simulink model "FLIGHT_Hexacopter_V2_1"  (R2024a)
settings: Solver=FixedStepDiscrete  StartTime=0.0  StopTime=inf  FixedStep=SampleTime_SAS  RelTol=1e-3  EnableMultiTasking=on
InitFcn:
  | Init_FLIGHT_Hexacopter
values from neighbouring files (symbols this model uses):
  d2r = pi/180    (= 0.0174532925199)    [Init_FLIGHT_Hexacopter.m]
  Jxx = 0.0211    [Init_FLIGHT_Hexacopter.m]
  Jyy = 0.0219    [Init_FLIGHT_Hexacopter.m]
  Jzz = 0.0366    [Init_FLIGHT_Hexacopter.m]
  Kpp = 3.3894    [Init_FLIGHT_Hexacopter_fromNCMS.m]
  Kpr = 3.3894    [Init_FLIGHT_Hexacopter_fromNCMS.m]
  MAX_CONTROL_ANGLE_PITCH = 30*pi/180    (= 0.523598775598)    [Init_FLIGHT_Hexacopter.m]    (also in Init_FLIGHT_Hexacopter_fromNCMS.m = 0.349065850399)
  MAX_CONTROL_ANGLE_RATE_PITCH = 360*pi/180    (= 6.28318530718)    [Init_FLIGHT_Hexacopter.m]    (also in Init_FLIGHT_Hexacopter_fromNCMS.m)
  MAX_CONTROL_ANGLE_RATE_ROLL = 360*pi/180    (= 6.28318530718)    [Init_FLIGHT_Hexacopter.m]    (also in Init_FLIGHT_Hexacopter_fromNCMS.m)
  MAX_CONTROL_ANGLE_RATE_Y = 120*pi/180    (= 2.09439510239)    [Init_FLIGHT_Hexacopter.m]    (also in Init_FLIGHT_Hexacopter_fromNCMS.m)
  MAX_CONTROL_ANGLE_ROLL = 30*pi/180    (= 0.523598775598)    [Init_FLIGHT_Hexacopter.m]    (also in Init_FLIGHT_Hexacopter_fromNCMS.m = 0.349065850399)
  MAX_CONTROL_VELOCITY_XY = 1.5    [Init_FLIGHT_Hexacopter.m]    (also in Init_FLIGHT_Hexacopter_fromNCMS.m)
  MAX_CONTROL_VELOCITY_Z = 1    [Init_FLIGHT_Hexacopter.m]    (also in Init_FLIGHT_Hexacopter_fromNCMS.m)
  SampleTime = 1/250    (= 0.004)    [Init_FLIGHT_Hexacopter.m]    (also in Init_FLIGHT_Hexacopter_fromNCMS.m = 0.01)
  SampleTime_SAS = 1/1000    (= 0.001)    [Init_FLIGHT_Hexacopter.m]
undefined symbols (not defined in the file or in its folder): arguments, DiscIntNeverNeededParam, event_sequence, id, log_levels, MPC_Z_D, MPC_Z_I, MPC_Z_P, timestamp
libraries: px4lib x42, simulink x9, px4Utilslib x8, px4uORBlib x8, slpidlib x5, simulink_extras x2, sharedtransform x1, px4Sensorslib x1, matrix_library x1
(part 2 of 3)

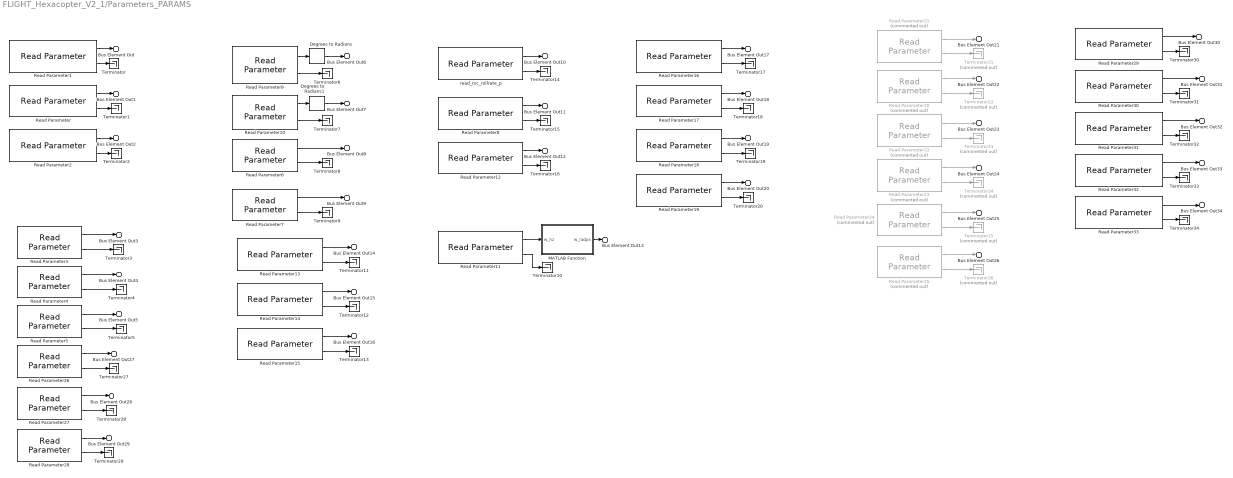
== system FLIGHT_Hexacopter_V2_1/Parameters_PARAMS ==
  Degrees to Radians : simulink_extras/Transformations/Degrees to Radians
  Degrees to Radians1 : simulink_extras/Transformations/Degrees to Radians
  MATLAB Function : MATLAB Function  TreatAsAtomicUnit=on
  Read Parameter : px4lib/Read Parameter  ParameterName=DOUBLET_DT  DataType=FLOAT  SampleTime=SampleTime
      settings: SourceProductName=UAV Toolbox Support Package for PX4 Autopilots
  Read Parameter1 : px4lib/Read Parameter  ParameterName=DOUBLET_PEAK_ANG  DataType=FLOAT  SampleTime=SampleTime
      settings: SourceProductName=UAV Toolbox Support Package for PX4 Autopilots
  Read Parameter10 : px4lib/Read Parameter  ParameterName=MC_PITCHRATE_MAX  DataType=FLOAT  SampleTime=SampleTime
      settings: SourceProductName=UAV Toolbox Support Package for PX4 Autopilots
  Read Parameter11 : px4lib/Read Parameter  ParameterName=IMU_DGYRO_CUTOFF  DataType=FLOAT  SampleTime=SampleTime
      settings: SourceProductName=UAV Toolbox Support Package for PX4 Autopilots
  Read Parameter12 : px4lib/Read Parameter  ParameterName=MC_ROLLRATE_D  DataType=FLOAT  SampleTime=SampleTime
      settings: SourceProductName=UAV Toolbox Support Package for PX4 Autopilots
  Read Parameter13 : px4lib/Read Parameter  ParameterName=MC_PITCHRATE_P  DataType=FLOAT  SampleTime=SampleTime
      settings: SourceProductName=UAV Toolbox Support Package for PX4 Autopilots
  Read Parameter14 : px4lib/Read Parameter  ParameterName=MC_PITCHRATE_I  DataType=FLOAT  SampleTime=SampleTime
      settings: SourceProductName=UAV Toolbox Support Package for PX4 Autopilots
  Read Parameter15 : px4lib/Read Parameter  ParameterName=MC_PITCHRATE_D  DataType=FLOAT  SampleTime=SampleTime
      settings: SourceProductName=UAV Toolbox Support Package for PX4 Autopilots
  Read Parameter16 : px4lib/Read Parameter  ParameterName=MC_YAWRATE_P  DataType=FLOAT  SampleTime=SampleTime
      settings: SourceProductName=UAV Toolbox Support Package for PX4 Autopilots
  Read Parameter17 : px4lib/Read Parameter  ParameterName=MC_YAWRATE_I  DataType=FLOAT  SampleTime=SampleTime
      settings: SourceProductName=UAV Toolbox Support Package for PX4 Autopilots
  Read Parameter18 : px4lib/Read Parameter  ParameterName=MC_YAWRATE_D  DataType=FLOAT  SampleTime=SampleTime
      settings: SourceProductName=UAV Toolbox Support Package for PX4 Autopilots
  Read Parameter19 : px4lib/Read Parameter  ParameterName=MC_YAWRATE_FF  DataType=FLOAT  SampleTime=SampleTime
      settings: SourceProductName=UAV Toolbox Support Package for PX4 Autopilots
  Read Parameter2 : px4lib/Read Parameter  ParameterName=DOUBLET_AXIS  DataType=INT32  SampleTime=SampleTime
      settings: SourceProductName=UAV Toolbox Support Package for PX4 Autopilots
  Read Parameter20 : px4lib/Read Parameter  Commented=on  ParameterName=FDD_M2_STATUS  DataType=INT32  SampleTime=SampleTime
      settings: SourceProductName=UAV Toolbox Support Package for PX4 Autopilots
  Read Parameter21 : px4lib/Read Parameter  Commented=on  ParameterName=FDD_M1_STATUS  DataType=INT32  SampleTime=SampleTime
      settings: SourceProductName=UAV Toolbox Support Package for PX4 Autopilots
  Read Parameter22 : px4lib/Read Parameter  Commented=on  ParameterName=FDD_M3_STATUS  DataType=INT32  SampleTime=SampleTime
      settings: SourceProductName=UAV Toolbox Support Package for PX4 Autopilots
  Read Parameter23 : px4lib/Read Parameter  Commented=on  ParameterName=FDD_M4_STATUS  DataType=INT32  SampleTime=SampleTime
      settings: SourceProductName=UAV Toolbox Support Package for PX4 Autopilots
  Read Parameter24 : px4lib/Read Parameter  Commented=on  ParameterName=FDD_M5_STATUS  DataType=INT32  SampleTime=SampleTime
      settings: SourceProductName=UAV Toolbox Support Package for PX4 Autopilots
  Read Parameter25 : px4lib/Read Parameter  Commented=on  ParameterName=FDD_M6_STATUS  DataType=INT32  SampleTime=SampleTime
      settings: SourceProductName=UAV Toolbox Support Package for PX4 Autopilots
  Read Parameter26 : px4lib/Read Parameter  ParameterName=MPC_THR_HOVER  DataType=FLOAT  SampleTime=SampleTime
      settings: SourceProductName=UAV Toolbox Support Package for PX4 Autopilots
  Read Parameter27 : px4lib/Read Parameter  ParameterName=MPC_XY_P  DataType=FLOAT  SampleTime=SampleTime
      settings: SourceProductName=UAV Toolbox Support Package for PX4 Autopilots
  Read Parameter28 : px4lib/Read Parameter  ParameterName=MPC_XY_VEL_P_ACC  DataType=FLOAT  SampleTime=SampleTime
      settings: SourceProductName=UAV Toolbox Support Package for PX4 Autopilots
  Read Parameter29 : px4lib/Read Parameter  ParameterName=K_SMC_P  DataType=FLOAT  SampleTime=SampleTime
      settings: SourceProductName=UAV Toolbox Support Package for PX4 Autopilots
  Read Parameter3 : px4lib/Read Parameter  ParameterName=MPC_Z_VEL_P_ACC  DataType=FLOAT  SampleTime=SampleTime
      settings: SourceProductName=UAV Toolbox Support Package for PX4 Autopilots
  Read Parameter30 : px4lib/Read Parameter  ParameterName=K_SMC_I  DataType=FLOAT  SampleTime=SampleTime
      settings: SourceProductName=UAV Toolbox Support Package for PX4 Autopilots
  Read Parameter31 : px4lib/Read Parameter  ParameterName=K_SMC_D  DataType=FLOAT  SampleTime=SampleTime
      settings: SourceProductName=UAV Toolbox Support Package for PX4 Autopilots
  Read Parameter32 : px4lib/Read Parameter  ParameterName=K_REACH_S  DataType=FLOAT  SampleTime=SampleTime
      settings: SourceProductName=UAV Toolbox Support Package for PX4 Autopilots
  Read Parameter33 : px4lib/Read Parameter  ParameterName=K_REACH_P  DataType=FLOAT  SampleTime=SampleTime
      settings: SourceProductName=UAV Toolbox Support Package for PX4 Autopilots
  Read Parameter4 : px4lib/Read Parameter  ParameterName=MPC_Z_VEL_I_ACC  DataType=FLOAT  SampleTime=SampleTime
      settings: SourceProductName=UAV Toolbox Support Package for PX4 Autopilots
  Read Parameter5 : px4lib/Read Parameter  ParameterName=MPC_Z_VEL_D_ACC  DataType=FLOAT  SampleTime=SampleTime
      settings: SourceProductName=UAV Toolbox Support Package for PX4 Autopilots
  Read Parameter6 : px4lib/Read Parameter  ParameterName=MC_ROLL_P  DataType=FLOAT  SampleTime=SampleTime
      settings: SourceProductName=UAV Toolbox Support Package for PX4 Autopilots
  Read Parameter7 : px4lib/Read Parameter  ParameterName=MC_PITCH_P  DataType=FLOAT  SampleTime=SampleTime
      settings: SourceProductName=UAV Toolbox Support Package for PX4 Autopilots
  Read Parameter8 : px4lib/Read Parameter  ParameterName=MC_ROLLRATE_I  DataType=FLOAT  SampleTime=SampleTime
      settings: SourceProductName=UAV Toolbox Support Package for PX4 Autopilots
  Read Parameter9 : px4lib/Read Parameter  ParameterName=MC_ROLLRATE_MAX  DataType=FLOAT  SampleTime=SampleTime
      settings: SourceProductName=UAV Toolbox Support Package for PX4 Autopilots
  Terminator{,1..20,27..34} (29 alike) : Terminator
  Terminator{21..26} (6 alike) : Terminator  Commented=on
  read_mc_rollrate_p : px4lib/Read Parameter  ParameterName=MC_ROLLRATE_P  DataType=FLOAT  SampleTime=SampleTime
      settings: SourceProductName=UAV Toolbox Support Package for PX4 Autopilots
  Bus Element Out : Outport  PortName=PARAMS  Element=DOUBLET_PEAK_ANG
  Bus Element Out1 : Outport  PortName=PARAMS  Element=DOUBLET_DT
  Bus Element Out2 : Outport  PortName=PARAMS  Element=DOUBLET_AXIS
  Bus Element Out3 : Outport  PortName=PARAMS  Element=MPC_Z_VEL_P_ACC
  Bus Element Out4 : Outport  PortName=PARAMS  Element=MPC_Z_VEL_I_ACC
  Bus Element Out5 : Outport  PortName=PARAMS  Element=MPC_Z_VEL_D_ACC
  Bus Element Out6 : Outport  PortName=PARAMS  Element=MC_ROLLRATE_MAX
  Bus Element Out7 : Outport  PortName=PARAMS  Element=MC_PITCHRATE_MAX
  Bus Element Out8 : Outport  PortName=PARAMS  Element=MC_ROLL_P
  Bus Element Out9 : Outport  PortName=PARAMS  Element=MC_PITCH_P
  Bus Element Out10 : Outport  PortName=PARAMS  Element=MC_ROLLRATE_P
  Bus Element Out11 : Outport  PortName=PARAMS  Element=MC_ROLLRATE_I
  Bus Element Out12 : Outport  PortName=PARAMS  Element=MC_ROLLRATE_D
  Bus Element Out13 : Outport  PortName=PARAMS  Element=IMU_DGYRO_CUTOFF
  Bus Element Out14 : Outport  PortName=PARAMS  Element=MC_PITCHRATE_P
  Bus Element Out15 : Outport  PortName=PARAMS  Element=MC_PITCHRATE_I
  Bus Element Out16 : Outport  PortName=PARAMS  Element=MC_PITCHRATE_D
  Bus Element Out17 : Outport  PortName=PARAMS  Element=MC_YAWRATE_P
  Bus Element Out18 : Outport  PortName=PARAMS  Element=MC_YAWRATE_I
  Bus Element Out19 : Outport  PortName=PARAMS  Element=MC_YAWRATE_D
  Bus Element Out20 : Outport  PortName=PARAMS  Element=MC_YAWRATE_FF
  Bus Element Out21 : Outport  PortName=PARAMS  Element=FDD_M1_STATUS
  Bus Element Out22 : Outport  PortName=PARAMS  Element=FDD_M2_STATUS
  Bus Element Out23 : Outport  PortName=PARAMS  Element=FDD_M3_STATUS
  Bus Element Out24 : Outport  PortName=PARAMS  Element=FDD_M4_STATUS
  Bus Element Out25 : Outport  PortName=PARAMS  Element=FDD_M5_STATUS
  Bus Element Out26 : Outport  PortName=PARAMS  Element=FDD_M6_STATUS
  Bus Element Out27 : Outport  PortName=PARAMS  Element=MPC_THR_HOVER
  Bus Element Out28 : Outport  PortName=PARAMS  Element=MPC_XY_P
  Bus Element Out29 : Outport  PortName=PARAMS  Element=MPC_XY_VEL_P_ACC
  Bus Element Out30 : Outport  PortName=PARAMS  Element=K_SMC_P
  Bus Element Out31 : Outport  PortName=PARAMS  Element=K_SMC_I
  Bus Element Out32 : Outport  PortName=PARAMS  Element=K_SMC_D
  Bus Element Out33 : Outport  PortName=PARAMS  Element=K_REACH_S
  Bus Element Out34 : Outport  PortName=PARAMS  Element=K_REACH_P
  wires:
  Read Parameter9/2 -> Terminator6/1
  Read Parameter10/1 -> Degrees to Radians1/1
  Read Parameter9/1 -> Degrees to Radians/1
  Read Parameter10/2 -> Terminator7/1
  Read Parameter7/1 -> Bus Element Out9/1
  Read Parameter7/2 -> Terminator9/1
  Read Parameter6/1 -> Bus Element Out8/1
  Read Parameter6/2 -> Terminator8/1
  Read Parameter11/2 -> Terminator10/1
  Read Parameter11/1 -> MATLAB Function/1(w_hz)
  Read Parameter1/1 -> Bus Element Out/1
  Read Parameter1/2 -> Terminator/1
  Read Parameter2/1 -> Bus Element Out2/1
  Read Parameter2/2 -> Terminator2/1
  Read Parameter/2 -> Terminator1/1
  Read Parameter/1 -> Bus Element Out1/1
  Read Parameter3/1 -> Bus Element Out3/1
  Read Parameter4/1 -> Bus Element Out4/1
  Read Parameter5/1 -> Bus Element Out5/1
  Read Parameter3/2 -> Terminator3/1
  Read Parameter4/2 -> Terminator4/1
  Read Parameter5/2 -> Terminator5/1
  Degrees to Radians1/1 -> Bus Element Out7/1
  Degrees to Radians/1 -> Bus Element Out6/1
  read_mc_rollrate_p/1 -> Bus Element Out10/1
  Read Parameter8/1 -> Bus Element Out11/1
  Read Parameter12/1 -> Bus Element Out12/1
  MATLAB Function/1(w_radps) -> Bus Element Out13/1
  Read Parameter13/1 -> Bus Element Out14/1
  Read Parameter14/1 -> Bus Element Out15/1
  Read Parameter15/1 -> Bus Element Out16/1
  Read Parameter13/2 -> Terminator11/1
  Read Parameter14/2 -> Terminator12/1
  Read Parameter15/2 -> Terminator13/1
  read_mc_rollrate_p/2 -> Terminator14/1
  Read Parameter8/2 -> Terminator15/1
  Read Parameter12/2 -> Terminator16/1
  Read Parameter16/1 -> Bus Element Out17/1
  Read Parameter17/1 -> Bus Element Out18/1
  Read Parameter18/1 -> Bus Element Out19/1
  Read Parameter19/1 -> Bus Element Out20/1
  Read Parameter16/2 -> Terminator17/1
  Read Parameter17/2 -> Terminator18/1
  Read Parameter18/2 -> Terminator19/1
  Read Parameter19/2 -> Terminator20/1
  Read Parameter21/1 -> Bus Element Out21/1
  Read Parameter20/1 -> Bus Element Out22/1
  Read Parameter22/1 -> Bus Element Out23/1
  Read Parameter23/1 -> Bus Element Out24/1
  Read Parameter24/1 -> Bus Element Out25/1
  Read Parameter25/1 -> Bus Element Out26/1
  Read Parameter21/2 -> Terminator21/1
  Read Parameter20/2 -> Terminator22/1
  Read Parameter22/2 -> Terminator23/1
  Read Parameter23/2 -> Terminator24/1
  Read Parameter24/2 -> Terminator25/1
  Read Parameter25/2 -> Terminator26/1
  Read Parameter26/1 -> Bus Element Out27/1
  Read Parameter26/2 -> Terminator27/1
  Read Parameter27/1 -> Bus Element Out28/1
  Read Parameter27/2 -> Terminator28/1
  Read Parameter28/1 -> Bus Element Out29/1
  Read Parameter28/2 -> Terminator29/1
  Read Parameter32/1 -> Bus Element Out33/1
  Read Parameter33/2 -> Terminator34/1
  Read Parameter31/2 -> Terminator32/1
  Read Parameter33/1 -> Bus Element Out34/1
  Read Parameter29/1 -> Bus Element Out30/1
  Read Parameter30/2 -> Terminator31/1
  Read Parameter30/1 -> Bus Element Out31/1
  Read Parameter32/2 -> Terminator33/1
  Read Parameter31/1 -> Bus Element Out32/1
  Read Parameter29/2 -> Terminator30/1

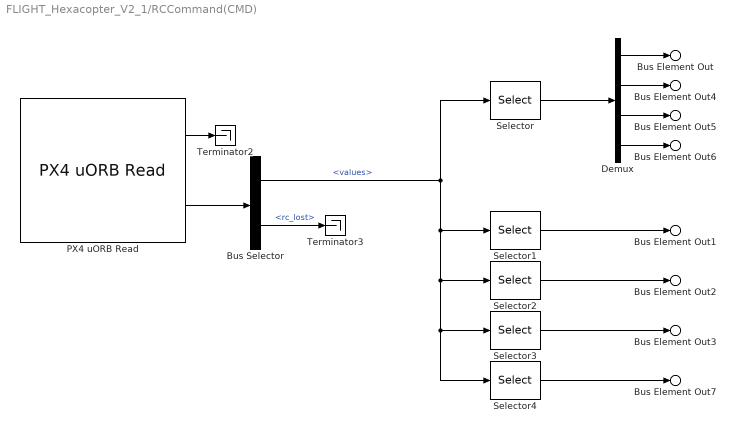
== system FLIGHT_Hexacopter_V2_1/RCCommand(CMD) ==
  Bus Selector : BusSelector  OutputSignals=values,rc_lost
  Demux : Demux
  PX4 uORB Read : px4uORBlib/PX4 uORB Read  uORBTopic=InputRc  selectInstance=InputRc  SampleTime=SampleTime  BlockingMode=off  BlockTimeout=1e-3
      settings: SourceProductName=PX4 uORB Read and Write Blocks
  Selector : Selector  InputPortWidth=18  IndexOptions=Index vector (dialog)  Indices=[1 2 4 3]  OutputSizes=1
  Selector1 : Selector  InputPortWidth=18  IndexOptions=Index vector (dialog)  Indices=[6]  OutputSizes=1
  Selector2 : Selector  InputPortWidth=18  IndexOptions=Index vector (dialog)  Indices=7  OutputSizes=1
  Selector3 : Selector  InputPortWidth=18  IndexOptions=Index vector (dialog)  Indices=8  OutputSizes=1
  Selector4 : Selector  InputPortWidth=18  IndexOptions=Index vector (dialog)  Indices=10  OutputSizes=1
  Terminator2 : Terminator
  Terminator3 : Terminator
  Bus Element Out : Outport  PortName=CMD  Element=rc_roll
  Bus Element Out1 : Outport  PortName=CMD  Element=rc_mode
  Bus Element Out2 : Outport  PortName=CMD  Element=rc_doublet
  Bus Element Out3 : Outport  PortName=CMD  Element=rc_inject_failure
  Bus Element Out4 : Outport  PortName=CMD  Element=rc_pitch
  Bus Element Out5 : Outport  PortName=CMD  Element=rc_yaw
  Bus Element Out6 : Outport  PortName=CMD  Element=rc_throttle
  Bus Element Out7 : Outport  PortName=CMD  Element=rc_ctrl_switch
  wires:
  Selector/1 -> Demux/1
  PX4 uORB Read/2 -> Bus Selector/1
  Bus Selector/2 -> Terminator3/1  "<rc_lost>"
  Selector1/1 -> Bus Element Out1/1
  Bus Selector/1 -> Selector4/1, Selector3/1, Selector2/1, Selector1/1, Selector/1  "<values>"
  PX4 uORB Read/1 -> Terminator2/1
  Demux/1 -> Bus Element Out/1
  Demux/2 -> Bus Element Out4/1
  Demux/3 -> Bus Element Out5/1
  Demux/4 -> Bus Element Out6/1
  Selector2/1 -> Bus Element Out2/1
  Selector3/1 -> Bus Element Out3/1
  Selector4/1 -> Bus Element Out7/1

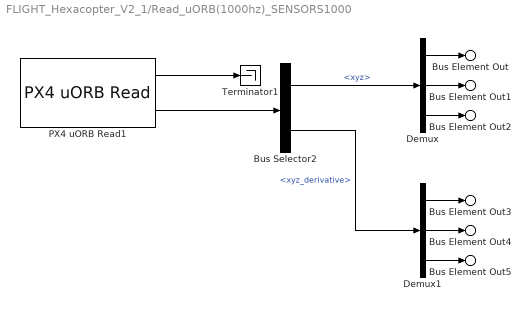
== system FLIGHT_Hexacopter_V2_1/Read_uORB(1000hz)_SENSORS1000 ==
  Bus Selector2 : BusSelector  OutputSignals=xyz,xyz_derivative
  Demux : Demux  Outputs=3
  Demux1 : Demux  Outputs=3
  PX4 uORB Read1 : px4uORBlib/PX4 uORB Read  uORBTopic=VehicleAngularVelocity  selectInstance=vehicle_angular_velocity  SampleTime=SampleTime_SAS  BlockingMode=off  BlockTimeout=1e-3
      settings: SourceProductName=PX4 uORB Read and Write Blocks
  Terminator1 : Terminator
  Bus Element Out : Outport  PortName=SENSORS1000  Element=P
  Bus Element Out1 : Outport  PortName=SENSORS1000  Element=Q
  Bus Element Out2 : Outport  PortName=SENSORS1000  Element=R
  Bus Element Out3 : Outport  PortName=SENSORS1000  Element=P_dot
  Bus Element Out4 : Outport  PortName=SENSORS1000  Element=Q_dot
  Bus Element Out5 : Outport  PortName=SENSORS1000  Element=R_dot
  wires:
  Bus Selector2/1 -> Demux/1  "<xyz>"
  PX4 uORB Read1/1 -> Terminator1/1
  Bus Selector2/2 -> Demux1/1  "<xyz_derivative>"
  PX4 uORB Read1/2 -> Bus Selector2/1
  Demux/1 -> Bus Element Out/1
  Demux/2 -> Bus Element Out1/1
  Demux/3 -> Bus Element Out2/1
  Demux1/1 -> Bus Element Out3/1
  Demux1/2 -> Bus Element Out4/1
  Demux1/3 -> Bus Element Out5/1

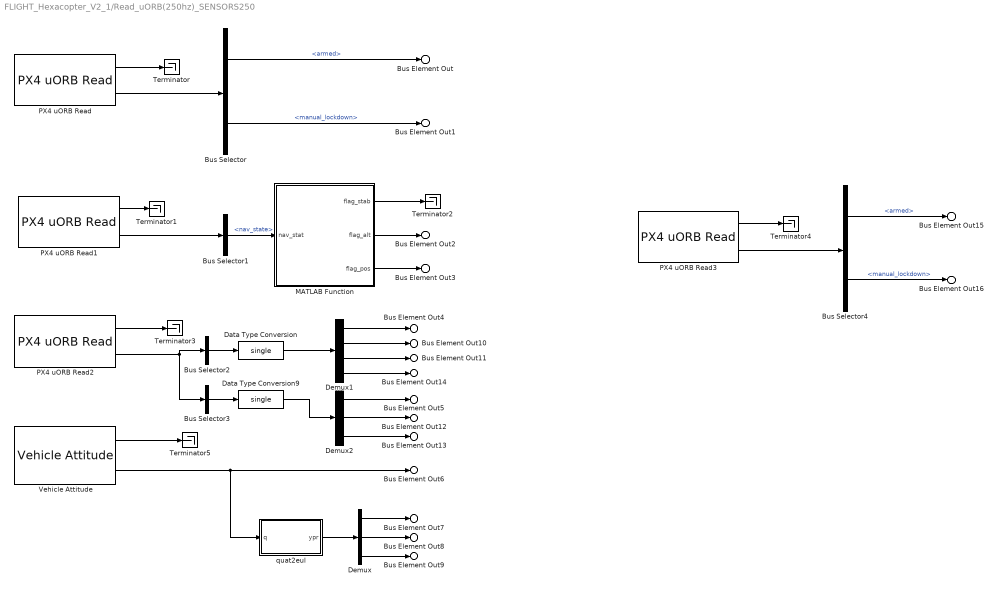
== system FLIGHT_Hexacopter_V2_1/Read_uORB(250hz)_SENSORS250 ==
  Bus Selector : BusSelector  OutputSignals=armed,manual_lockdown
  Bus Selector1 : BusSelector  OutputSignals=nav_state
  Bus Selector2 : BusSelector  OutputSignals=x,y,z,heading  OutputAsBus=on
  Bus Selector3 : BusSelector  OutputSignals=vx,vy,vz  OutputAsBus=on
  Bus Selector4 : BusSelector  OutputSignals=armed,manual_lockdown
  Data Type Conversion : DataTypeConversion  OutDataTypeStr=single  SaturateOnIntegerOverflow=off  RndMeth=Floor
  Data Type Conversion9 : DataTypeConversion  OutDataTypeStr=single  SaturateOnIntegerOverflow=off  RndMeth=Floor
  Demux : Demux  Outputs=3
  Demux1 : Demux
  Demux2 : Demux  Outputs=3
  MATLAB Function : MATLAB Function  TreatAsAtomicUnit=on
  PX4 uORB Read : px4uORBlib/PX4 uORB Read  uORBTopic=ActuatorArmed  selectInstance=ActuatorArmed  SampleTime=SampleTime  BlockingMode=off  BlockTimeout=1e-3
      settings: SourceProductName=PX4 uORB Read and Write Blocks
  PX4 uORB Read1 : px4uORBlib/PX4 uORB Read  uORBTopic=VehicleStatus  selectInstance=VehicleStatus  SampleTime=SampleTime  BlockingMode=off  BlockTimeout=1e-3
      settings: SourceProductName=PX4 uORB Read and Write Blocks
  PX4 uORB Read2 : px4uORBlib/PX4 uORB Read  uORBTopic=VehicleLocalPosition  selectInstance=vehicle_local_position  SampleTime=SampleTime  BlockingMode=off  BlockTimeout=1e-3
      settings: SourceProductName=PX4 uORB Read and Write Blocks
  PX4 uORB Read3 : px4uORBlib/PX4 uORB Read  uORBTopic=ActuatorArmed  selectInstance=ActuatorArmed  SampleTime=SampleTime  BlockingMode=off  BlockTimeout=1e-3
      settings: SourceProductName=PX4 uORB Read and Write Blocks
  Terminator{,1..5} (6 alike) : Terminator
  Vehicle Attitude : px4Sensorslib/Vehicle Attitude  rollRate=off  pitchRate=off  yawRate=off  quaternion=on  uorbTimeStamp=off  BlockingMode=off  BlockTimeout=0.001  sampleTime=SampleTime
  quat2eul : MATLAB Function  TreatAsAtomicUnit=on
  Bus Element Out : Outport  PortName=SENSORS250  Element=VehicleStatus_armed
  Bus Element Out1 : Outport  PortName=SENSORS250  Element=VehicleStatus_emergency_kill
  Bus Element Out2 : Outport  PortName=SENSORS250  Element=VehicleStatus_flag_altitude_mode
  Bus Element Out3 : Outport  PortName=SENSORS250  Element=VehicleStatus_flag_position_mode
  Bus Element Out4 : Outport  PortName=SENSORS250  Element=X
  Bus Element Out5 : Outport  PortName=SENSORS250  Element=U
  Bus Element Out6 : Outport  PortName=SENSORS250  Element=State_quaternion
  Bus Element Out7 : Outport  PortName=SENSORS250  Element=Psi
  Bus Element Out8 : Outport  PortName=SENSORS250  Element=Theta
  Bus Element Out9 : Outport  PortName=SENSORS250  Element=Phi
  Bus Element Out12 : Outport  PortName=SENSORS250  Element=V
  Bus Element Out13 : Outport  PortName=SENSORS250  Element=W
  Bus Element Out10 : Outport  PortName=SENSORS250  Element=Y
  Bus Element Out11 : Outport  PortName=SENSORS250  Element=Z
  Bus Element Out14 : Outport  PortName=SENSORS250  Element=Heading
  Bus Element Out15 : Outport  PortName=SENSORS250  Element=VehicleStatus_flag_armed
  Bus Element Out16 : Outport  PortName=SENSORS250  Element=VehicleStatus_flag_kill
  wires:
  Bus Selector/2 -> Bus Element Out1/1  "<manual_lockdown>"
  Bus Selector/1 -> Bus Element Out/1  "<armed>"
  PX4 uORB Read/1 -> Terminator/1
  PX4 uORB Read/2 -> Bus Selector/1
  PX4 uORB Read1/1 -> Terminator1/1
  PX4 uORB Read1/2 -> Bus Selector1/1
  MATLAB Function/3(flag_pos) -> Bus Element Out3/1
  Bus Selector1/1 -> MATLAB Function/1(nav_stat)  "<nav_state>"
  MATLAB Function/2(flag_alt) -> Bus Element Out2/1
  MATLAB Function/1(flag_stab) -> Terminator2/1
  Bus Selector3/1 -> Data Type Conversion9/1
  PX4 uORB Read2/1 -> Terminator3/1
  Bus Selector2/1 -> Data Type Conversion/1
  Vehicle Attitude/1 -> Terminator5/1
  PX4 uORB Read2/2 -> Bus Selector3/1, Bus Selector2/1
  Vehicle Attitude/2 -> quat2eul/1(q), Bus Element Out6/1
  quat2eul/1(ypr) -> Demux/1
  Demux/1 -> Bus Element Out7/1
  Demux/2 -> Bus Element Out8/1
  Demux/3 -> Bus Element Out9/1
  Data Type Conversion/1 -> Demux1/1
  Demux1/1 -> Bus Element Out4/1
  Demux1/2 -> Bus Element Out10/1
  Demux1/3 -> Bus Element Out11/1
  Data Type Conversion9/1 -> Demux2/1
  Demux2/1 -> Bus Element Out5/1
  Demux2/2 -> Bus Element Out12/1
  Demux2/3 -> Bus Element Out13/1
  Demux1/4 -> Bus Element Out14/1
  PX4 uORB Read3/2 -> Bus Selector4/1
  PX4 uORB Read3/1 -> Terminator4/1
  Bus Selector4/2 -> Bus Element Out16/1  "<manual_lockdown>"
  Bus Selector4/1 -> Bus Element Out15/1  "<armed>"

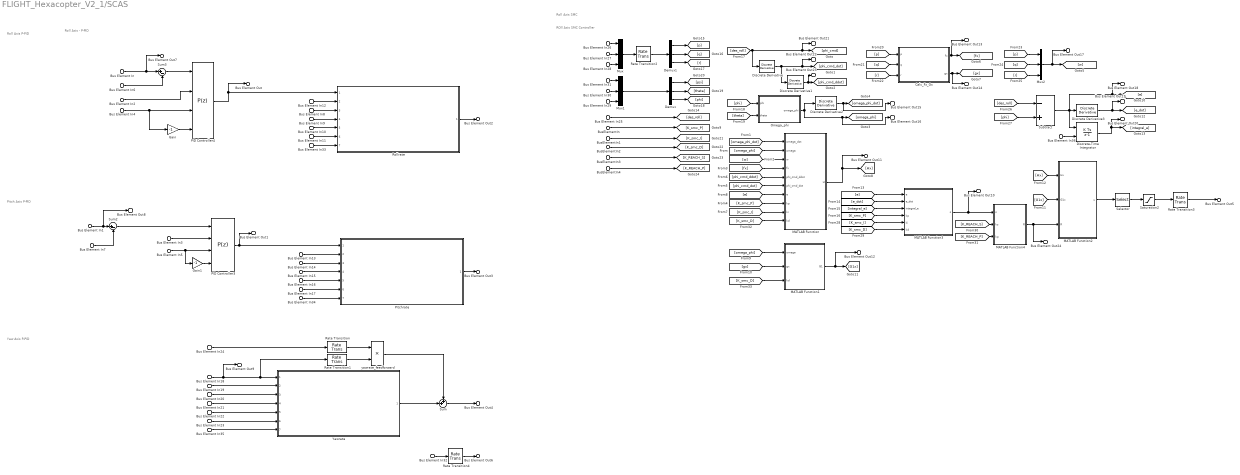
== system FLIGHT_Hexacopter_V2_1/SCAS ==
  note: Roll Axis P-PID
  note: Roll Axis - P-PID
  note: ROll Axis SMC Controller
  note: Pitch Axis P-PID
  note: Yaw Axis P-PID
  note: Roll Axis SMC
  Bus Element In : Inport  PortName=OFP  Element=des_roll
  Bus Element In25 : Inport  PortName=OFP  Element=des_roll
  Bus Element In1 : Inport  PortName=OFP  Element=des_pitch
  Bus Element In18 : Inport  PortName=OFP  Element=des_yr
  Bus Element In32 : Inport  PortName=OFP  Element=des_thr
  Bus Element In2 : Inport  Port=2  PortName=PARAMS  Element=MC_ROLL_P
  Bus Element In3 : Inport  Port=2  PortName=PARAMS  Element=MC_PITCH_P
  Bus Element In4 : Inport  Port=2  PortName=PARAMS  Element=MC_ROLLRATE_MAX
  Bus Element In5 : Inport  Port=2  PortName=PARAMS  Element=MC_PITCHRATE_MAX
  Bus Element In8 : Inport  Port=2  PortName=PARAMS  Element=MC_ROLLRATE_P
  Bus Element In9 : Inport  Port=2  PortName=PARAMS  Element=MC_ROLLRATE_I
  Bus Element In10 : Inport  Port=2  PortName=PARAMS  Element=MC_ROLLRATE_D
  Bus Element In11 : Inport  Port=2  PortName=PARAMS  Element=IMU_DGYRO_CUTOFF
  Bus Element In17 : Inport  Port=2  PortName=PARAMS  Element=IMU_DGYRO_CUTOFF
  Bus Element In23 : Inport  Port=2  PortName=PARAMS  Element=IMU_DGYRO_CUTOFF
  Bus Element In14 : Inport  Port=2  PortName=PARAMS  Element=MC_PITCHRATE_P
  Bus Element In15 : Inport  Port=2  PortName=PARAMS  Element=MC_PITCHRATE_I
  Bus Element In16 : Inport  Port=2  PortName=PARAMS  Element=MC_PITCHRATE_D
  Bus Element In20 : Inport  Port=2  PortName=PARAMS  Element=MC_YAWRATE_P
  Bus Element In21 : Inport  Port=2  PortName=PARAMS  Element=MC_YAWRATE_I
  Bus Element In22 : Inport  Port=2  PortName=PARAMS  Element=MC_YAWRATE_D
  Bus Element In24 : Inport  Port=2  PortName=PARAMS  Element=MC_YAWRATE_FF
  BusElementIn : Inport  Port=2  PortName=PARAMS  Element=K_SMC_P
  BusElementIn1 : Inport  Port=2  PortName=PARAMS  Element=K_SMC_I
  BusElementIn2 : Inport  Port=2  PortName=PARAMS  Element=K_SMC_D
  BusElementIn3 : Inport  Port=2  PortName=PARAMS  Element=K_REACH_S
  BusElementIn4 : Inport  Port=2  PortName=PARAMS  Element=K_REACH_P
  Bus Element In6 : Inport  Port=3  PortName=SENSORS250  Element=Phi
  Bus Element In29 : Inport  Port=3  PortName=SENSORS250  Element=Phi
  Bus Element In7 : Inport  Port=3  PortName=SENSORS250  Element=Theta
  Bus Element In30 : Inport  Port=3  PortName=SENSORS250  Element=Theta
  Bus Element In31 : Inport  Port=3  PortName=SENSORS250  Element=Psi
  Bus Element In{33..36} (4 alike) : Inport  Port=3  PortName=SENSORS250  Element=VehicleStatus_flag_armed
  Bus Element In12 : Inport  Port=4  PortName=SENSORS1000  Element=P
  Bus Element In26 : Inport  Port=4  PortName=SENSORS1000  Element=P
  Bus Element In13 : Inport  Port=4  PortName=SENSORS1000  Element=Q
  Bus Element In27 : Inport  Port=4  PortName=SENSORS1000  Element=Q
  Bus Element In19 : Inport  Port=4  PortName=SENSORS1000  Element=R
  Bus Element In28 : Inport  Port=4  PortName=SENSORS1000  Element=R
  Calc_Fx_Gx : Subsystem
  Demux : Demux  Outputs=3
  Demux1 : Demux  Outputs=3
  Discrete Derivative{,1..3} (4 alike) : simulink/Discrete/Discrete Derivative  gainval=1.0  ICPrevScaledInput=0.0  OutMin=[]  OutMax=[]  OutDataType=fixdt(1, 16)  OutScaling=2^-10  DoSatur=off
  Discrete-Time Integrator : DiscreteIntegrator  ExternalReset=rising  SampleTime=-1  ICPrevOutput=DiscIntNeverNeededParam  ICPrevScaledInput=DiscIntNeverNeededParam
  Gain : Gain  Gain=-1
  Gain1 : Gain  Gain=-1
  MATLAB Function : MATLAB Function  TreatAsAtomicUnit=on
  MATLAB Function1 : MATLAB Function  TreatAsAtomicUnit=on
  MATLAB Function2 : MATLAB Function  TreatAsAtomicUnit=on
  MATLAB Function3 : MATLAB Function  TreatAsAtomicUnit=on
  MATLAB Function4 : MATLAB Function  TreatAsAtomicUnit=on
  Mux : Mux  Inputs=3
  Mux1 : Mux  Inputs=3
  Mux2 : Mux  Inputs=3
  Omega_phi : MATLAB Function  TreatAsAtomicUnit=on
  PID Controller3 : slpidlib/PID Controller  Controller=P  Form=Parallel  TimeDomain=Discrete-time  UseExternalTs=off  SampleTime=SampleTime  IntegratorMethod=Forward Euler  FilterMethod=Forward Euler  ControllerParametersSource=external  P=Kpp  I=1  UseKiTs=off  D=0  UseExternalDerivativeSource=off  N=100  UseFilter=on  TunerSelectOption=Transfer Function Based (PID Tuner App)  InitialConditionSource=internal  InitialConditionForIntegrator=0  InitialConditionForFilter=0  DifferentiatorICPrevScaledInput=0  ExternalReset=none  TrackingMode=off  Kt=1  LimitOutput=on  SatLimitsSource=external  UpperSaturationLimit=MAX_CONTROL_ANGLE_RATE_PITCH  LowerSaturationLimit=-MAX_CONTROL_ANGLE_RATE_PITCH  LinearizeAsGain=on  AntiWindupMode=none  Kb=1  LimitIntegrator=off  UpperIntegratorSaturationLimit=inf  LowerIntegratorSaturationLimit=-inf  POutMin=[]  POutMax=[]  IOutMin=[]  IOutMax=[]  DOutMin=[]  DOutMax=[]  NOutMin=[]  NOutMax=[]  SumOutMin=[]  SumOutMax=[]  SaturationOutMin=[]  SaturationOutMax=[]  PParamMin=[]  PParamMax=[]  IParamMin=[]  IParamMax=[]  DParamMin=[]  DParamMax=[]  NParamMin=[]  NParamMax=[]  KbParamMin=[]  KbParamMax=[]  KtParamMin=[]  KtParamMax=[]  KbOutMin=[]  KbOutMax=[]  KtOutMin=[]  KtOutMax=[]  IntegratorOutMin=[]  IntegratorOutMax=[]  FilterOutMin=[]  FilterOutMax=[]  SumI1OutMin=[]  SumI1OutMax=[]  SumI2OutMin=[]  SumI2OutMax=[]  SumI3OutMin=[]  SumI3OutMax=[]  SumI4OutMin=[]  SumI4OutMax=[]  SumDOutMin=[]  SumDOutMax=[]  DifferentiatorOutMin=[]  DifferentiatorOutMax=[]  FilterDiffOutCoefMin=[]  FilterDiffOutCoefMax=[]  ReciprocalOutMin=[]  ReciprocalOutMax=[]  SumDenOutMin=[]  SumDenOutMax=[]  SumNumOutMin=[]  SumNumOutMax=[]  DivideOutMin=[]  DivideOutMax=[]  UdiffTsProdOutMin=[]  UdiffTsProdOutMax=[]  NTsProdOutMin=[]  NTsProdOutMax=[]  UintegralTsProdOutMin=[]  UintegralTsProdOutMax=[]  UngainTsProdOutMin=[]  UngainTsProdOutMax=[]  ClampingZeroOutDataTypeStr=Inherit: Inherit via back propagation  ClampingZeroOutMin=[]  ClampingZeroOutMax=[]  FilterDenConstantOutDataTypeStr=Inherit: Inherit via back propagation  FilterDenConstantOutMin=[]  FilterDenConstantOutMax=[]  PCopyOutDataTypeStr=Inherit: Inherit via back propagation  PCopyOutMin=[]  PCopyOutMax=[]  NCopyOutDataTypeStr=Inherit: Inherit via back propagation  NCopyOutMin=[]  NCopyOutMax=[]  IntegratorContinuousStateAttributes=''  IntegratorStateMustResolveToSignalObject=off  IntegratorRTWStateStorageClass=Auto  FilterContinuousStateAttributes=''  FilterStateMustResolveToSignalObject=off  FilterRTWStateStorageClass=Auto  ParallelPVariant=ExternalParameters  IdealPVariant=Disabled  IVariant=Disabled  DVariant=Disabled  IntegratorVariant=Disabled  SatVariant=External  AWVariant=Disabled  PCopyVariant=Disabled  TRVariant=Disabled  FdbkBlocksVariant=Forward  IdealPFdbkVariant=Disabled  SatFdbkVariant=Disabled  DerivativeFilterVariant=Disabled  NVariant=Disabled  NCopyVariant=Disabled_SignalSpec  FilterICVariant=Disabled  IntegratorICVariant=Disabled  ExternalResetVariant=Disabled  TRSumVariant=Passthrough  SumFdbkVariant=Disabled  SumVariant=Passthrough_P  TsampFilterVariant=InternalTs  TsampNgainVariant=Passthrough  TsampIntegralVariant=Disabled_SignalSpec  ExternalSaturationOutDataTypeStr=Inherit: Same as second input  DerivativeSourceVariant=Disabled
  PID Controller4 : slpidlib/PID Controller  Controller=P  Form=Parallel  TimeDomain=Discrete-time  UseExternalTs=off  SampleTime=SampleTime  IntegratorMethod=Forward Euler  FilterMethod=Forward Euler  ControllerParametersSource=external  P=Kpr  I=1  UseKiTs=off  D=0  UseExternalDerivativeSource=off  N=100  UseFilter=on  TunerSelectOption=Transfer Function Based (PID Tuner App)  InitialConditionSource=internal  InitialConditionForIntegrator=0  InitialConditionForFilter=0  DifferentiatorICPrevScaledInput=0  ExternalReset=none  TrackingMode=off  Kt=1  LimitOutput=on  SatLimitsSource=external  UpperSaturationLimit=MAX_CONTROL_ANGLE_RATE_ROLL  LowerSaturationLimit=-MAX_CONTROL_ANGLE_RATE_ROLL  LinearizeAsGain=on  AntiWindupMode=none  Kb=1  LimitIntegrator=off  UpperIntegratorSaturationLimit=inf  LowerIntegratorSaturationLimit=-inf  POutMin=[]  POutMax=[]  IOutMin=[]  IOutMax=[]  DOutMin=[]  DOutMax=[]  NOutMin=[]  NOutMax=[]  SumOutMin=[]  SumOutMax=[]  SaturationOutMin=[]  SaturationOutMax=[]  PParamMin=[]  PParamMax=[]  IParamMin=[]  IParamMax=[]  DParamMin=[]  DParamMax=[]  NParamMin=[]  NParamMax=[]  KbParamMin=[]  KbParamMax=[]  KtParamMin=[]  KtParamMax=[]  KbOutMin=[]  KbOutMax=[]  KtOutMin=[]  KtOutMax=[]  IntegratorOutMin=[]  IntegratorOutMax=[]  FilterOutMin=[]  FilterOutMax=[]  SumI1OutMin=[]  SumI1OutMax=[]  SumI2OutMin=[]  SumI2OutMax=[]  SumI3OutMin=[]  SumI3OutMax=[]  SumI4OutMin=[]  SumI4OutMax=[]  SumDOutMin=[]  SumDOutMax=[]  DifferentiatorOutMin=[]  DifferentiatorOutMax=[]  FilterDiffOutCoefMin=[]  FilterDiffOutCoefMax=[]  ReciprocalOutMin=[]  ReciprocalOutMax=[]  SumDenOutMin=[]  SumDenOutMax=[]  SumNumOutMin=[]  SumNumOutMax=[]  DivideOutMin=[]  DivideOutMax=[]  UdiffTsProdOutMin=[]  UdiffTsProdOutMax=[]  NTsProdOutMin=[]  NTsProdOutMax=[]  UintegralTsProdOutMin=[]  UintegralTsProdOutMax=[]  UngainTsProdOutMin=[]  UngainTsProdOutMax=[]  ClampingZeroOutDataTypeStr=Inherit: Inherit via back propagation  ClampingZeroOutMin=[]  ClampingZeroOutMax=[]  FilterDenConstantOutDataTypeStr=Inherit: Inherit via back propagation  FilterDenConstantOutMin=[]  FilterDenConstantOutMax=[]  PCopyOutDataTypeStr=Inherit: Inherit via back propagation  PCopyOutMin=[]  PCopyOutMax=[]  NCopyOutDataTypeStr=Inherit: Inherit via back propagation  NCopyOutMin=[]  NCopyOutMax=[]  IntegratorContinuousStateAttributes=''  IntegratorStateMustResolveToSignalObject=off  IntegratorRTWStateStorageClass=Auto  FilterContinuousStateAttributes=''  FilterStateMustResolveToSignalObject=off  FilterRTWStateStorageClass=Auto  ParallelPVariant=ExternalParameters  IdealPVariant=Disabled  IVariant=Disabled  DVariant=Disabled  IntegratorVariant=Disabled  SatVariant=External  AWVariant=Disabled  PCopyVariant=Disabled  TRVariant=Disabled  FdbkBlocksVariant=Forward  IdealPFdbkVariant=Disabled  SatFdbkVariant=Disabled  DerivativeFilterVariant=Disabled  NVariant=Disabled  NCopyVariant=Disabled_SignalSpec  FilterICVariant=Disabled  IntegratorICVariant=Disabled  ExternalResetVariant=Disabled  TRSumVariant=Passthrough  SumFdbkVariant=Disabled  SumVariant=Passthrough_P  TsampFilterVariant=InternalTs  TsampNgainVariant=Passthrough  TsampIntegralVariant=Disabled_SignalSpec  ExternalSaturationOutDataTypeStr=Inherit: Same as second input  DerivativeSourceVariant=Disabled
  Pitchrate : Subsystem  ReferencedSubsystem=SAS_PI_slash_D_Controller
  Rate Transition{,1,3..4} (4 alike) : RateTransition  OutPortSampleTime=SampleTime_SAS
  Rate Transition2 : RateTransition  OutPortSampleTime=SampleTime
  Rollrate : Subsystem  ReferencedSubsystem=SAS_PI_slash_D_Controller
  Saturation2 : Saturate  UpperLimit=1  LowerLimit=-1
  Selector : Selector  InputPortWidth=3  IndexOptions=Index vector (dialog)  Indices=1  OutputSizes=1
  Subtract : Sum  Inputs=-+
  Sum : Sum  Inputs=++|
  Sum2 : Sum  Inputs=|+-
  Sum3 : Sum  Inputs=|+-
  Yawrate : Subsystem  ReferencedSubsystem=SAS_PI_slash_D_Controller
  yawrate_feedforward : Product
  Bus Element Out : Outport  PortName=SCAS  Element=des_rollrate
  Bus Element Out1 : Outport  PortName=SCAS  Element=des_pitchrate
  Bus Element Out2 : Outport  PortName=SCAS  Element=tau_roll
  Bus Element Out3 : Outport  PortName=SCAS  Element=tau_pitch
  Bus Element Out4 : Outport  PortName=SCAS  Element=tau_yaw
  Bus Element Out5 : Outport  PortName=SCAS  Element=tau_roll_smc
  Bus Element Out6 : Outport  PortName=SCAS  Element=tau_throttle
  Bus Element Out7 : Outport  PortName=SCAS  Element=des_roll
  Bus Element Out8 : Outport  PortName=SCAS  Element=des_pitch
  Bus Element Out9 : Outport  PortName=SCAS  Element=des_yr
  Bus Element Out10 : Outport  PortName=SCAS  Element=smc_s
  Bus Element Out11 : Outport  PortName=SCAS  Element=smc_hx
  Bus Element Out12 : Outport  PortName=SCAS  Element=smc_g1x
  Bus Element Out13 : Outport  PortName=SCAS  Element=smc_fx
  Bus Element Out14 : Outport  PortName=SCAS  Element=smc_gx
  Bus Element Out15 : Outport  PortName=SCAS  Element=smc_omega_phi_dot
  Bus Element Out16 : Outport  PortName=SCAS  Element=smc_omega_phi
  Bus Element Out17 : Outport  PortName=SCAS  Element=smc_omega
  Bus Element Out18 : Outport  PortName=SCAS  Element=smc_e
  Bus Element Out19 : Outport  PortName=SCAS  Element=smc_e_dot
  Bus Element Out20 : Outport  PortName=SCAS  Element=smc_integral_e
  Bus Element Out21 : Outport  PortName=SCAS  Element=smc_phi_cmd
  Bus Element Out22 : Outport  PortName=SCAS  Element=smc_phi_cmd_dot
  Bus Element Out23 : Outport  PortName=SCAS  Element=smc_phi_cmd_ddot
  Bus Element Out24 : Outport  PortName=SCAS  Element=smc_r
  wires:
  Bus Element In4/1 -> Gain/1, PID Controller4/3
  Gain/1 -> PID Controller4/4
  Bus Element In3/1 -> PID Controller3/2
  Bus Element In/1 -> Bus Element Out7/1, Sum3/1
  Sum2/1 -> PID Controller3/1
  Gain1/1 -> PID Controller3/4
  Bus Element In2/1 -> PID Controller4/2
  Sum3/1 -> PID Controller4/1
  Bus Element In5/1 -> Gain1/1, PID Controller3/3
  Bus Element In1/1 -> Bus Element Out8/1, Sum2/1
  Bus Element In6/1 -> Sum3/2
  Bus Element In7/1 -> Sum2/2
  PID Controller4/1 -> Rollrate/1, Bus Element Out/1
  Bus Element In8/1 -> Rollrate/3
  Bus Element In9/1 -> Rollrate/4
  Bus Element In10/1 -> Rollrate/5
  Bus Element In11/1 -> Rollrate/6
  Bus Element In12/1 -> Rollrate/2
  PID Controller3/1 -> Pitchrate/1, Bus Element Out1/1
  Bus Element In17/1 -> Pitchrate/6
  Bus Element In16/1 -> Pitchrate/5
  Bus Element In15/1 -> Pitchrate/4
  Bus Element In14/1 -> Pitchrate/3
  Bus Element In13/1 -> Pitchrate/2
  Bus Element In23/1 -> Yawrate/6
  Bus Element In18/1 -> Bus Element Out9/1, Rate Transition1/1, Yawrate/1
  Bus Element In19/1 -> Yawrate/2
  Bus Element In20/1 -> Yawrate/3
  Bus Element In21/1 -> Yawrate/4
  Bus Element In22/1 -> Yawrate/5
  yawrate_feedforward/1 -> Sum/1
  Bus Element In24/1 -> Rate Transition/1
  Yawrate/1 -> Sum/2
  Sum/1 -> Bus Element Out4/1
  Pitchrate/1 -> Bus Element Out3/1
  Rollrate/1 -> Bus Element Out2/1
  Rate Transition/1 -> yawrate_feedforward/1
  Rate Transition1/1 -> yawrate_feedforward/2
  Mux/1 -> Rate Transition2/1
  Bus Element In26/1 -> Mux/1
  Bus Element In27/1 -> Mux/2
  Bus Element In28/1 -> Mux/3
  Bus Element In30/1 -> Mux1/2
  Bus Element In31/1 -> Mux1/1
  Bus Element In29/1 -> Mux1/3
  Bus Element In32/1 -> Rate Transition4/1
  Rate Transition4/1 -> Bus Element Out6/1
  Bus Element In33/1 -> Rollrate/7
  Bus Element In34/1 -> Pitchrate/7
  Bus Element In35/1 -> Yawrate/7
  [K_smc_D] -> MATLAB Function1/3(kd)
  [omega_phi] -> MATLAB Function/2(omega)
  Discrete Derivative1/1 -> Bus Element Out23/1, [phi_cmd_ddot]
  Discrete-Time Integrator/1 -> Bus Element Out20/1, [integral_e]
  [G1x] -> MATLAB Function2/2(G1x)
  [K_smc_D] -> MATLAB Function3/6(kd)
  [des_roll] -> Subtract/1
  MATLAB Function1/1(G1) -> Bus Element Out12/1, [G1x]
  [K_smc_I] -> MATLAB Function/9(ki)
  [e_dot] -> MATLAB Function3/2(e_dot)
  [p] -> Mux2/1
  Subtract/1 -> Discrete-Time Integrator/1, Discrete Derivative3/1, Bus Element Out18/1, [e]
  [gx] -> MATLAB Function1/2(gx)
  [K_REACH_S] -> MATLAB Function4/2(ks)
  [Hx] -> MATLAB Function2/1(Hx)
  [integral_e] -> MATLAB Function3/3(integral_e)
  Omega_phi/1(omega_phi) -> Discrete Derivative2/1, Bus Element Out16/1, [omega_phi]
  Calc_Fx_Gx/1(fx) -> Bus Element Out13/1, [fx]
  [des_roll] -> Discrete Derivative/1, Bus Element Out21/1, [phi_cmd]
  [K_smc_P] -> MATLAB Function3/4(kp)
  Discrete Derivative/1 -> Discrete Derivative1/1, Bus Element Out22/1, [phi_cmd_dot]
  [theta] -> Omega_phi/2(theta)
  [q] -> Calc_Fx_Gx/2(q)
  [w] -> MATLAB Function/3(w)
  [K_REACH_P] -> MATLAB Function4/3(kp)
  MATLAB Function3/1(s) -> Bus Element Out10/1, MATLAB Function4/1(s)
  MATLAB Function4/1(R) -> Bus Element Out24/1, MATLAB Function2/3(R)
  [omega_phi_dot] -> MATLAB Function/1(omega_dot)
  [K_smc_I] -> MATLAB Function3/5(ki)
  [p] -> Calc_Fx_Gx/1(p)
  Calc_Fx_Gx/2(gx) -> Bus Element Out14/1, [gx]
  Saturation2/1 -> Rate Transition3/1
  [r] -> Calc_Fx_Gx/3(r)
  [q] -> Mux2/2
  Mux2/1 -> Bus Element Out17/1, [w]
  [K_smc_D] -> MATLAB Function/10(kd)
  Selector/1 -> Saturation2/1
  [phi] -> Subtract/2
  MATLAB Function2/1(u) -> Selector/1
  [fx] -> MATLAB Function/4(fx)
  [K_smc_P] -> MATLAB Function/8(kp)
  [phi_cmd_dot] -> MATLAB Function/6(phi_cmd_dot)
  [phi_cmd_ddot] -> MATLAB Function/5(phi_cmd_ddot)
  Discrete Derivative2/1 -> Bus Element Out15/1, [omega_phi_dot]
  [e] -> MATLAB Function/7(e)
  MATLAB Function/1(H) -> Bus Element Out11/1, [Hx]
  Discrete Derivative3/1 -> Bus Element Out19/1, [e_dot]
  [e] -> MATLAB Function3/1(e)
  [omega_phi] -> MATLAB Function1/1(omega)
  [phi] -> Omega_phi/1(phi)
  [r] -> Mux2/3
  Mux1/1 -> Demux/1
  Demux1/3 -> [r]
  Demux1/1 -> [p]
  Demux/3 -> [phi]
  Demux1/2 -> [q]
  Bus Element In25/1 -> [des_roll]
  Demux/2 -> [theta]
  Rate Transition2/1 -> Demux1/1
  Demux/1 -> [psi]
  BusElementIn/1 -> [K_smc_P]
  BusElementIn1/1 -> [K_smc_I]
  BusElementIn2/1 -> [K_smc_D]
  BusElementIn3/1 -> [K_REACH_S]
  BusElementIn4/1 -> [K_REACH_P]
  Rate Transition3/1 -> Bus Element Out5/1
  Bus Element In36/1 -> Discrete-Time Integrator/2

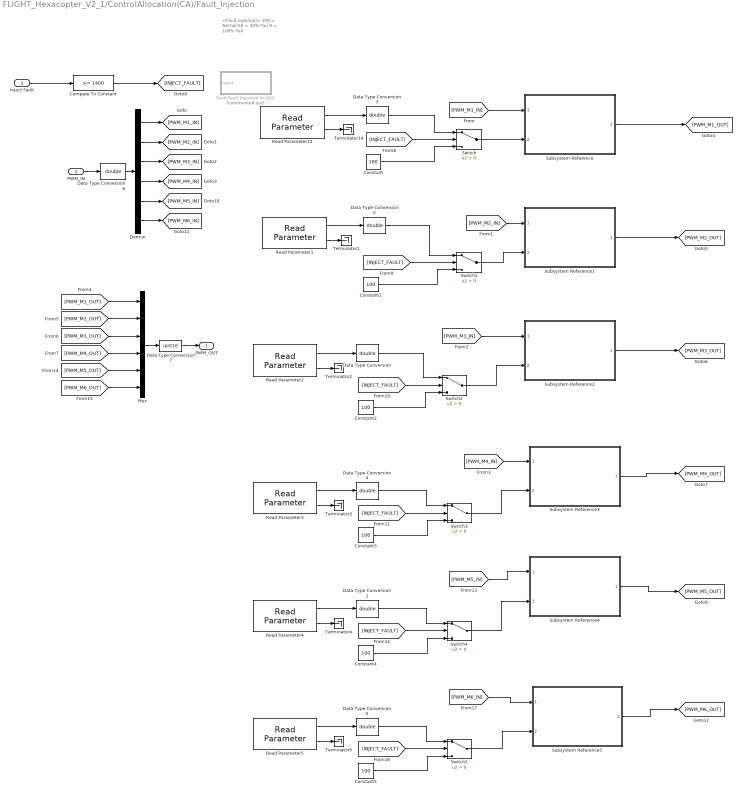
== system FLIGHT_Hexacopter_V2_1/ControlAllocation(CA)/Fault_Injection ==
  note: <Fault Injection>
      | 100 = Nornal
      | 50 = 50% Fail
      | 0 = 100% Fail
  PWM_IN : Inport
  Inject Fault : Inport  Port=2
  Compare To Constant : simulink/Logic and Bit Operations/Compare To Constant  relop=>=  const=1400  OutDataTypeStr=boolean
  Constant{,1..5} (6 alike) : Constant  Value=100
  Data Type Conversion{,1..6} (7 alike) : DataTypeConversion  OutDataTypeStr=double  SaturateOnIntegerOverflow=off  RndMeth=Floor
  Data Type Conversion7 : DataTypeConversion  OutDataTypeStr=uint16  SaturateOnIntegerOverflow=off  RndMeth=Floor
  Demux : Demux  Outputs=6
  Mux : Mux  Inputs=6
  Read Parameter1 : px4lib/Read Parameter  ParameterName=FDD_M2_STATUS  DataType=INT32  SampleTime=SampleTime_SAS
      settings: SourceProductName=UAV Toolbox Support Package for PX4 Autopilots
  Read Parameter13 : px4lib/Read Parameter  ParameterName=FDD_M1_STATUS  DataType=INT32  SampleTime=SampleTime_SAS
      settings: SourceProductName=UAV Toolbox Support Package for PX4 Autopilots
  Read Parameter2 : px4lib/Read Parameter  ParameterName=FDD_M3_STATUS  DataType=INT32  SampleTime=SampleTime_SAS
      settings: SourceProductName=UAV Toolbox Support Package for PX4 Autopilots
  Read Parameter3 : px4lib/Read Parameter  ParameterName=FDD_M4_STATUS  DataType=INT32  SampleTime=SampleTime_SAS
      settings: SourceProductName=UAV Toolbox Support Package for PX4 Autopilots
  Read Parameter4 : px4lib/Read Parameter  ParameterName=FDD_M5_STATUS  DataType=INT32  SampleTime=SampleTime_SAS
      settings: SourceProductName=UAV Toolbox Support Package for PX4 Autopilots
  Read Parameter5 : px4lib/Read Parameter  ParameterName=FDD_M6_STATUS  DataType=INT32  SampleTime=SampleTime_SAS
      settings: SourceProductName=UAV Toolbox Support Package for PX4 Autopilots
  Send Fault Injection to QGC : Subsystem  Commented=on  TreatAsAtomicUnit=on
  Subsystem Reference{,1..5} (6 alike) : Subsystem  ReferencedSubsystem=calculate_fault_injected_pwm
  Switch{,1..5} (6 alike) : Switch  Criteria=u2 > Threshold  SaturateOnIntegerOverflow=off  InputSameDT=off
  Terminator{1..5,14} (6 alike) : Terminator
  PWM_OUT : Outport
  wires:
  Read Parameter13/2 -> Terminator14/1
  Read Parameter1/2 -> Terminator1/1
  Read Parameter2/2 -> Terminator2/1
  Read Parameter2/1 -> Data Type Conversion/1
  Read Parameter3/2 -> Terminator3/1
  Read Parameter3/1 -> Data Type Conversion4/1
  Read Parameter13/1 -> Data Type Conversion3/1
  Read Parameter1/1 -> Data Type Conversion2/1
  Demux/1 -> [PWM_M1_IN]
  Demux/2 -> [PWM_M2_IN]
  Demux/3 -> [PWM_M3_IN]
  Demux/4 -> [PWM_M4_IN]
  Mux/1 -> Data Type Conversion7/1
  [PWM_M1_OUT] -> Mux/1
  [PWM_M2_OUT] -> Mux/2
  [PWM_M3_OUT] -> Mux/3
  [PWM_M4_OUT] -> Mux/4
  Inject Fault/1 -> Compare To Constant/1
  Compare To Constant/1 -> [INJECT_FAULT]
  Data Type Conversion3/1 -> Switch/1
  [INJECT_FAULT] -> Switch/2
  Constant/1 -> Switch/3
  Constant1/1 -> Switch1/3
  [INJECT_FAULT] -> Switch1/2
  Constant2/1 -> Switch2/3
  [INJECT_FAULT] -> Switch2/2
  Data Type Conversion/1 -> Switch2/1
  Constant3/1 -> Switch3/3
  [INJECT_FAULT] -> Switch3/2
  Data Type Conversion4/1 -> Switch3/1
  Read Parameter4/1 -> Data Type Conversion1/1
  Data Type Conversion1/1 -> Switch4/1
  Constant4/1 -> Switch4/3
  Read Parameter4/2 -> Terminator4/1
  [INJECT_FAULT] -> Switch4/2
  Demux/5 -> [PWM_M5_IN]
  Demux/6 -> [PWM_M6_IN]
  [PWM_M5_OUT] -> Mux/5
  [PWM_M6_OUT] -> Mux/6
  Data Type Conversion5/1 -> Switch5/1
  Read Parameter5/2 -> Terminator5/1
  [INJECT_FAULT] -> Switch5/2
  Read Parameter5/1 -> Data Type Conversion5/1
  Constant5/1 -> Switch5/3
  Data Type Conversion2/1 -> Switch1/1
  [PWM_M1_IN] -> Subsystem Reference/1
  Switch/1 -> Subsystem Reference/2
  [PWM_M2_IN] -> Subsystem Reference1/1
  Switch1/1 -> Subsystem Reference1/2
  [PWM_M3_IN] -> Subsystem Reference2/1
  Switch2/1 -> Subsystem Reference2/2
  Switch3/1 -> Subsystem Reference3/2
  [PWM_M4_IN] -> Subsystem Reference3/1
  [PWM_M5_IN] -> Subsystem Reference4/1
  Switch4/1 -> Subsystem Reference4/2
  [PWM_M6_IN] -> Subsystem Reference5/1
  Switch5/1 -> Subsystem Reference5/2
  Subsystem Reference/1 -> [PWM_M1_OUT]
  Subsystem Reference1/1 -> [PWM_M2_OUT]
  Subsystem Reference2/1 -> [PWM_M3_OUT]
  Subsystem Reference3/1 -> [PWM_M4_OUT]
  Subsystem Reference4/1 -> [PWM_M5_OUT]
  Subsystem Reference5/1 -> [PWM_M6_OUT]
  Data Type Conversion6/1 -> Demux/1
  PWM_IN/1 -> Data Type Conversion6/1
  Data Type Conversion7/1 -> PWM_OUT/1

== system FLIGHT_Hexacopter_V2_1/Logging/Normalize_pwm6 ==
  In1 : Inport
  Constant : Constant  Value=1000  OutDataTypeStr=single  SampleTime=SampleTime_SAS
  Gain : Gain  Gain=1/1000
  Saturation : Saturate  UpperLimit=2000  LowerLimit=1000
  Subtract : Sum  Inputs=+-
  Out1 : Outport
  wires:
  In1/1 -> Saturation/1
  Saturation/1 -> Subtract/1
  Constant/1 -> Subtract/2
  Subtract/1 -> Gain/1
  Gain/1 -> Out1/1

== system FLIGHT_Hexacopter_V2_1/OFP/NED2Body1 ==
  NED : Inport
  Heading : Inport  Port=2
  Calculate Transformation Matrix : Subsystem
  MatrixMultiply : Product  Multiplication=Matrix(*)
  BODY : Outport
  wires:
  Calculate Transformation Matrix/1(R) -> MatrixMultiply/1
  Heading/1 -> Calculate Transformation Matrix/1(theta)
  NED/1 -> MatrixMultiply/2
  MatrixMultiply/1 -> BODY/1

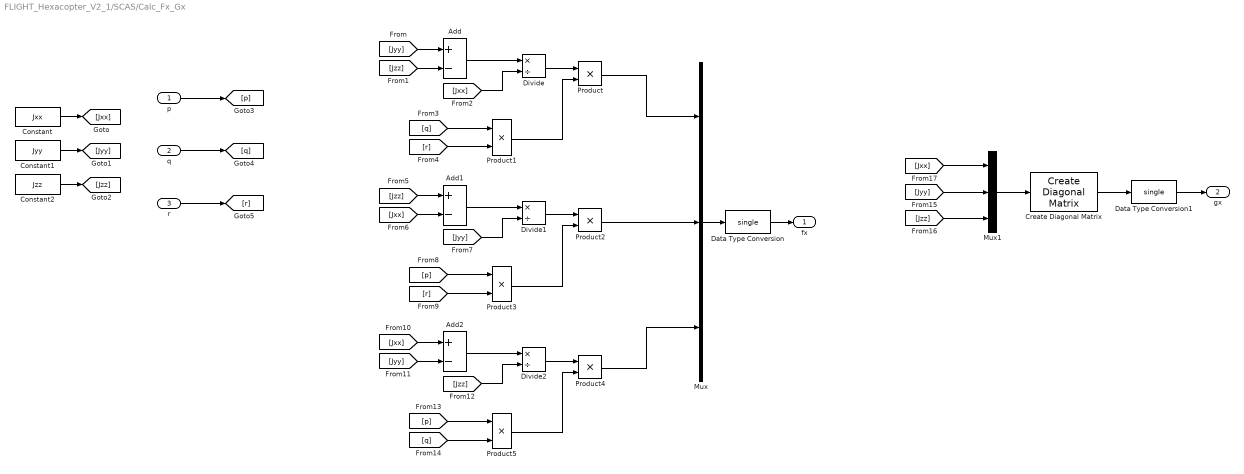
== system FLIGHT_Hexacopter_V2_1/SCAS/Calc_Fx_Gx ==
  p : Inport
  q : Inport  Port=2
  r : Inport  Port=3
  Add : Sum  Inputs=+-
  Add1 : Sum  Inputs=+-
  Add2 : Sum  Inputs=+-
  Constant : Constant  Value=Jxx  OutDataTypeStr=single
  Constant1 : Constant  Value=Jyy  OutDataTypeStr=single
  Constant2 : Constant  Value=Jzz  OutDataTypeStr=single
  Create Diagonal Matrix : matrix_library/Create Diagonal Matrix
  Data Type Conversion : DataTypeConversion  OutDataTypeStr=single  SaturateOnIntegerOverflow=off  RndMeth=Floor
  Data Type Conversion1 : DataTypeConversion  OutDataTypeStr=single  SaturateOnIntegerOverflow=off  RndMeth=Floor
  Divide : Product  Inputs=*/
  Divide1 : Product  Inputs=*/
  Divide2 : Product  Inputs=*/
  Mux : Mux  Inputs=3
  Mux1 : Mux  Inputs=3
  Product{,1..5} (6 alike) : Product
  fx : Outport
  gx : Outport  Port=2
  wires:
  Constant/1 -> [Jxx]
  Constant1/1 -> [Jyy]
  Constant2/1 -> [Jzz]
  [Jyy] -> Add/1
  [Jzz] -> Add/2
  Add/1 -> Divide/1
  [Jxx] -> Divide/2
  Divide/1 -> Product/1
  p/1 -> [p]
  q/1 -> [q]
  r/1 -> [r]
  [q] -> Product1/1
  [r] -> Product1/2
  Product1/1 -> Product/2
  Product/1 -> Mux/1
  [p] -> Product3/1
  Product2/1 -> Mux/2
  [r] -> Product3/2
  [Jzz] -> Add1/1
  Add1/1 -> Divide1/1
  Product3/1 -> Product2/2
  [Jxx] -> Add1/2
  Divide1/1 -> Product2/1
  [Jyy] -> Divide1/2
  [Jyy] -> Add2/2
  Divide2/1 -> Product4/1
  [Jxx] -> Add2/1
  Product5/1 -> Product4/2
  [q] -> Product5/2
  [p] -> Product5/1
  Add2/1 -> Divide2/1
  Product4/1 -> Mux/3
  [Jzz] -> Divide2/2
  Mux/1 -> Data Type Conversion/1
  [Jxx] -> Mux1/1
  [Jyy] -> Mux1/2
  [Jzz] -> Mux1/3
  Create Diagonal Matrix/1 -> Data Type Conversion1/1
  Mux1/1 -> Create Diagonal Matrix/1
  Data Type Conversion/1 -> fx/1
  Data Type Conversion1/1 -> gx/1

== system FLIGHT_Hexacopter_V2_1/ControlAllocation(CA)/Fault_Injection/Send Fault Injection to QGC ==
  Inject : Inport
  Bus Assignment : BusAssignment  AssignedSignals=timestamp,id,event_sequence,arguments,log_levels
  PX4 Timestamp : px4Utilslib/PX4 Timestamp  SampleTime=SampleTime
      settings: SourceProductName=PX4 Utility Blocks
  PX4 uORB Message : px4uORBlib/PX4 uORB Message  uORBTopic=Event  SampleTime=inf  selectInstance=Event
      settings: SourceProductName=PX4 uORB Read and Write Blocks
  PX4 uORB Write : px4uORBlib/PX4 uORB Write  uORBTopic=FailsafeFlags  selectInstance=FailsafeFlags  MessageQueueLen=1
      settings: SourceProductName=PX4 uORB Read and Write Blocks
  wires:
  PX4 uORB Message/1 -> Bus Assignment/1
  Bus Assignment/1 -> PX4 uORB Write/1
  PX4 Timestamp/1 -> Bus Assignment/2

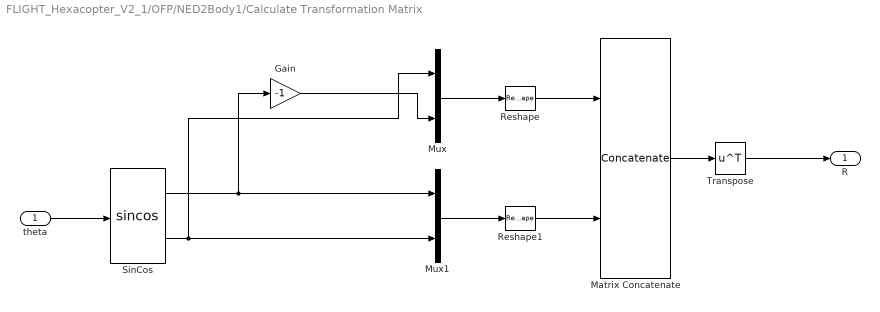
== system FLIGHT_Hexacopter_V2_1/OFP/NED2Body1/Calculate Transformation Matrix ==
  theta : Inport
  Gain : Gain  Gain=-1
  Matrix Concatenate : Concatenate  Mode=Multidimensional array
  Mux : Mux  Inputs=2
  Mux1 : Mux  Inputs=2
  Reshape : Reshape  OutputDimensionality=Row vector (2-D)
  Reshape1 : Reshape  OutputDimensionality=Row vector (2-D)
  SinCos : Trigonometry  Operator=sincos
  Transpose : Math  Operator=transpose
  R : Outport
  wires:
  Reshape1/1 -> Matrix Concatenate/2
  Reshape/1 -> Matrix Concatenate/1
  Transpose/1 -> R/1
  Matrix Concatenate/1 -> Transpose/1
  Mux1/1 -> Reshape1/1
  Mux/1 -> Reshape/1
  Gain/1 -> Mux/2
  SinCos/1 -> Mux1/1, Gain/1
  SinCos/2 -> Mux/1, Mux1/2
  theta/1 -> SinCos/1

== matlab function FLIGHT_Hexacopter_V2_1/SCAS/MATLAB Function3 ==
  data: e input; s output; e_dot input; integral_e input; kp input; ki input; kd input
function s = SlidingSurface(e, e_dot, integral_e, kp, ki, kd)

% PID Like Sliding Surface

s = kd*e_dot + kp*e + ki*integral_e;

== matlab function FLIGHT_Hexacopter_V2_1/SCAS/MATLAB Function4 ==
  data: s input; R output; ks input; kp input
function R = ReachingLaw(s, ks, kp)

R = -ks*sign(s) - kp*s;

== matlab function FLIGHT_Hexacopter_V2_1/SCAS/Omega_phi ==
  data: phi input; omega_phi output; theta input
function omega_phi  = CalcOmega(phi, theta)

omega_phi = [1, sin(phi)*tan(theta), cos(phi)*tan(theta)];

== matlab function FLIGHT_Hexacopter_V2_1/Parameters_PARAMS/MATLAB Function ==
  data: w_hz input; w_radps output
function w_radps= hz2radps(w_hz)

w_radps = w_hz * 2*pi;
